simulink model "Regulador_Sist_Segun_Orden"  (R2016a)
settings: Solver=VariableStepAuto  StartTime=0.0  StopTime=10.0  RelTol=1e-3
values from neighbouring files (symbols this model uses):
  K = [0 0 1][B AB A^2B]^-1phi(A)    phi(A)-->ec.deseada en term. de A    [Ecuaciones.m]
undefined symbols (not defined in the file or in its folder): A, B, C, K1, K2
settings Model: Creator=Daniel  LastModifiedBy=Daniel

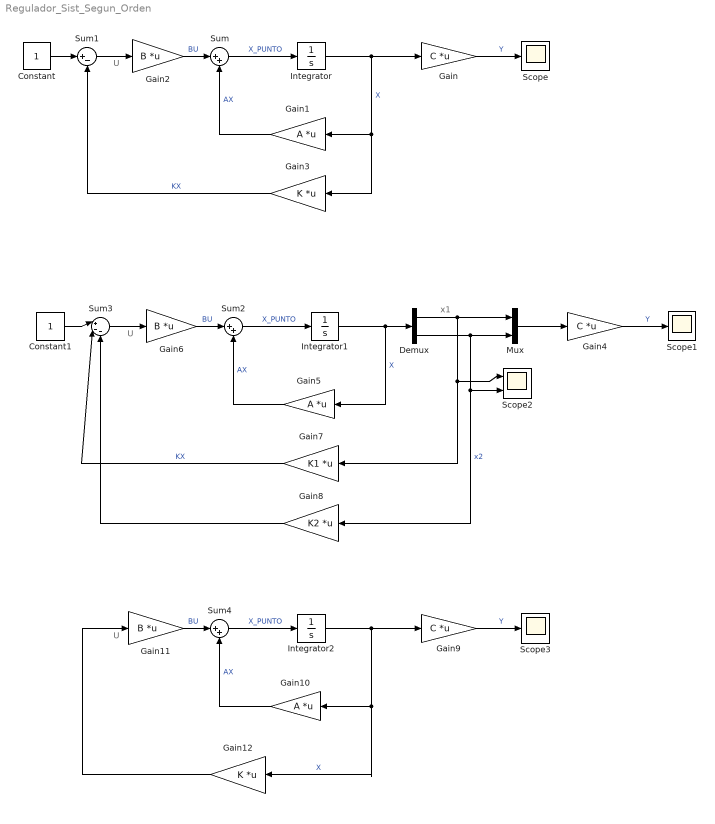
== system Regulador_Sist_Segun_Orden ==
  note: x1
  note: U
  note: U
  note: U
  Constant : Constant
  Constant1 : Constant
  Demux : Demux  Outputs=2
  Gain : Gain  Gain=C  Multiplication=Matrix(K*u) (u vector)
  Gain1 : Gain  Gain=A  Multiplication=Matrix(K*u) (u vector)
  Gain10 : Gain  Gain=A  Multiplication=Matrix(K*u) (u vector)
  Gain11 : Gain  Gain=B  Multiplication=Matrix(K*u) (u vector)
  Gain12 : Gain  Gain=K  Multiplication=Matrix(K*u) (u vector)
  Gain2 : Gain  Gain=B  Multiplication=Matrix(K*u) (u vector)
  Gain3 : Gain  Gain=K  Multiplication=Matrix(K*u) (u vector)
  Gain4 : Gain  Gain=C  Multiplication=Matrix(K*u) (u vector)
  Gain5 : Gain  Gain=A  Multiplication=Matrix(K*u) (u vector)
  Gain6 : Gain  Gain=B  Multiplication=Matrix(K*u) (u vector)
  Gain7 : Gain  Gain=K1  Multiplication=Matrix(K*u) (u vector)
  Gain8 : Gain  Gain=K2  Multiplication=Matrix(K*u) (u vector)
  Gain9 : Gain  Gain=C  Multiplication=Matrix(K*u) (u vector)
  Integrator : Integrator
  Integrator1 : Integrator
  Integrator2 : Integrator
  Mux : Mux  Inputs=2
  Scope : Scope
  Scope1 : Scope
  Scope2 : Scope  NumInputPorts=2
  Scope3 : Scope
  Sum : Sum  Inputs=|++
  Sum1 : Sum  Inputs=|+-
  Sum2 : Sum  Inputs=|++
  Sum3 : Sum  Inputs=|+--
  Sum4 : Sum  Inputs=|++
  wires:
  Sum/1 -> Integrator/1  "X_PUNTO"
  Integrator/1 -> Gain1/1, Gain3/1, Gain/1  "X"
  Gain1/1 -> Sum/2  "AX"
  Gain2/1 -> Sum/1  "BU"
  Gain3/1 -> Sum1/2  "KX"
  Sum1/1 -> Gain2/1
  Constant/1 -> Sum1/1
  Gain/1 -> Scope/1  "Y"
  Sum2/1 -> Integrator1/1  "X_PUNTO"
  Integrator1/1 -> Demux/1, Gain5/1  "X"
  Gain5/1 -> Sum2/2  "AX"
  Gain6/1 -> Sum2/1  "BU"
  Gain7/1 -> Sum3/2  "KX"
  Sum3/1 -> Gain6/1
  Constant1/1 -> Sum3/1
  Gain4/1 -> Scope1/1  "Y"
  Demux/1 -> Mux/1, Scope2/1, Gain7/1
  Gain8/1 -> Sum3/3
  Demux/2 -> Mux/2, Gain8/1, Scope2/2  "x2"
  Mux/1 -> Gain4/1
  Sum4/1 -> Integrator2/1  "X_PUNTO"
  Integrator2/1 -> Gain9/1, Gain12/1, Gain10/1  "X"
  Gain10/1 -> Sum4/2  "AX"
  Gain11/1 -> Sum4/1  "BU"
  Gain9/1 -> Scope3/1  "Y"
  Gain12/1 -> Gain11/1
